simulink model "sensor_signal_chain"  (R2022a)
settings: Solver=ode45  StartTime=0.0  StopTime=12  RelTol=1e-6  AbsTol=1e-8
settings Model: Creator=HJL  LastModifiedBy=HJL

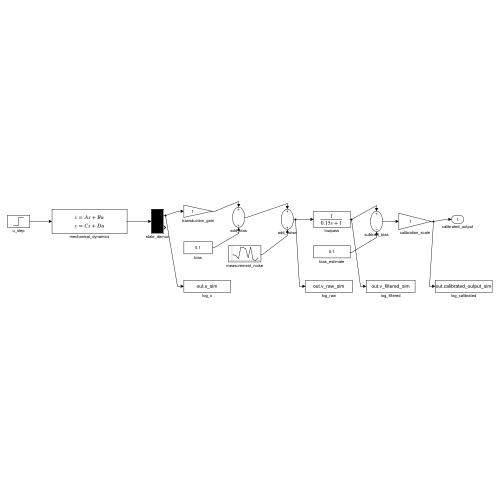
[thumbnail: Simulink's stored preview of the top-level diagram]
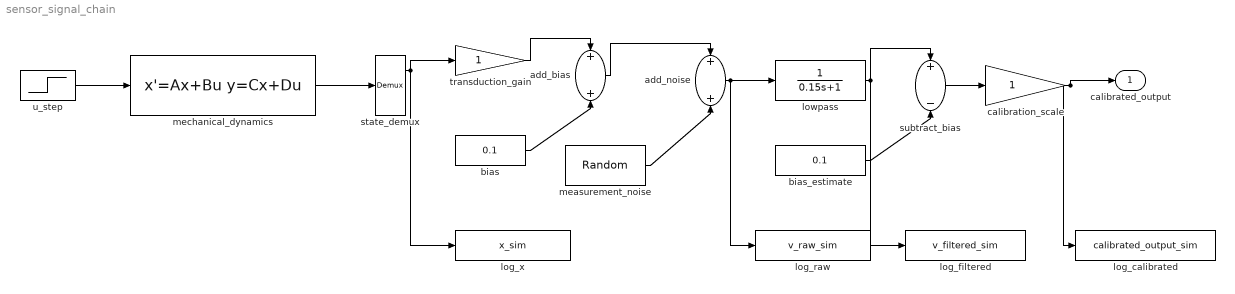
== system sensor_signal_chain ==
  add_bias : Sum
  add_noise : Sum
  bias : Constant  Value=0.1
  bias_estimate : Constant  Value=0.1
  calibration_scale : Gain
  log_calibrated : ToWorkspace  VariableName=calibrated_output_sim  SaveFormat=Timeseries  SampleTime=-1
  log_filtered : ToWorkspace  VariableName=v_filtered_sim  SaveFormat=Timeseries  SampleTime=-1
  log_raw : ToWorkspace  VariableName=v_raw_sim  SaveFormat=Timeseries  SampleTime=-1
  log_x : ToWorkspace  VariableName=x_sim  SaveFormat=Timeseries  SampleTime=-1
  lowpass : TransferFcn  Denominator=[0.15 1]
  measurement_noise : RandomNumber  Variance=0.0001  Seed=7  SampleTime=0.01
  mechanical_dynamics : StateSpace  A=[0 1; -1.2 -0.2]  B=[0; 1]  C=[1 0; 0 1]  D=[0; 0]  InitialCondition=[0; 0]
  state_demux : Demux  Outputs=2
  subtract_bias : Sum  Inputs=+-
  transduction_gain : Gain
  u_step : Step  SampleTime=0
  calibrated_output : Outport
  wires:
  u_step/1 -> mechanical_dynamics/1
  mechanical_dynamics/1 -> state_demux/1
  state_demux/1 -> transduction_gain/1, log_x/1
  transduction_gain/1 -> add_bias/1
  bias/1 -> add_bias/2
  add_bias/1 -> add_noise/1
  measurement_noise/1 -> add_noise/2
  add_noise/1 -> lowpass/1, log_raw/1
  lowpass/1 -> subtract_bias/1, log_filtered/1
  bias_estimate/1 -> subtract_bias/2
  subtract_bias/1 -> calibration_scale/1
  calibration_scale/1 -> calibrated_output/1, log_calibrated/1
